simulink model "exp11_2"  (R2019b)
settings: Solver=FixedStepAuto  StartTime=0.0  StopTime=10.0  FixedStep=0.01  RelTol=1e-3
settings Model: Creator=Sing Ngai  LastModifiedBy=Sing Ngai

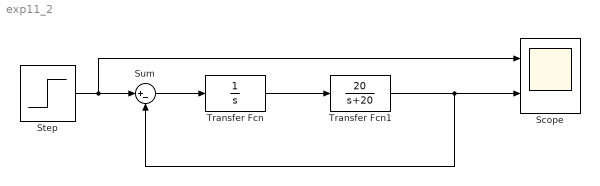
== system exp11_2 ==
  Scope : Scope  NumInputPorts=2
  Step : Step  Before=1  SampleTime=0
  Sum : Sum  Inputs=|+-
  Transfer Fcn : TransferFcn  Denominator=[1 0]
  Transfer Fcn1 : TransferFcn  Numerator=[20]  Denominator=[1 20]
  wires:
  Transfer Fcn/1 -> Transfer Fcn1/1
  Step/1 -> Scope/1, Sum/1
  Transfer Fcn1/1 -> Sum/2, Scope/2
  Sum/1 -> Transfer Fcn/1
